simulink model "IEEE80211a"  (Simulink 10.0)
settings: Solver=VariableStepDiscrete  StartTime=0.0  StopTime=inf  RelTol=1e-3  EnableMultiTasking=on
PreLoadFcn:
  | load IEEE80211a_init;
undefined symbols (not defined in the file): hyst, j, magnitude, params, QAM, thres
libraries: simulink x27, IEEE80211a_lib x19, dspsigops x19, dspmtrx3 x19, dspsigattribs x15, dspmlti3 x10, dspstat3 x6, dspmathops x5, dspindex x3, dspsrcs4 x3, dspbuff3 x2, dspxfrm3 x2
(part 2 of 2)

== system IEEE80211a/Multipath channel/Multipath Rayleigh Fading Channel2 ==
  In : Inport
  Multipath Fading Channel : Subsystem  mask(Multipath Fading Channel){Fd=Fd, LOSFd=0, K=0, simTs=simTs, delayVec=delayVec, gainVecdB=gainVecdB, normGain=on, Seed=Seed}
      mask prompts: Fd "Doppler frequency (Hz):"; LOSFd "Line-of-sight Doppler frequency (Hz):"; K "K-factor:"; simTs "Sample time (sec):"; delayVec "Delay vector (sec):"; gainVecdB "Gain vector (dB):"; normGain "Normalize gain vector to 0 dB overall gain"; Seed "Initial seed:"
      mask help:
      | Multipath fading channel for complex baseband signals.
      |
      | Multiplies the input signal with samples of a complex random process. The spectrum of the random process is given by the Jakes PSD, where the Doppler frequency parameter determines the maximum Doppler frequency. The K-factor parameter specifies the linear ratio of power in the direct path to the diffuse power.
      |
      | The number of paths equals the length of either the 'Delay vector' or 'Gain vector' parameters.
      mask init:
      | [ecode,emsg,params] = commblkfadingchan2(gcb,Fd,LOSFd,K,simTs,delayVec,gainVecdB,normGain,Seed);
      | if(ecode==1)
      |     error(emsg);
      | elseif(ecode==2)
      |     warning(emsg);
      | end;
      mask Display:
      | plot(0,0,100,100,[05 15 10 10 05 10 18 14 13 7.5 13 41 44 47 50 53 57 59 100-[13 7.5 13 14 18 10 5 10 10 15 5]],[70 70 70 85 92 85 79 82 90 88.5 90 90 87 93 87 93 87 90 90 88.5 90 82 79 85 92 85 70 70 70]);
      | disp('Multipath\nFading')
  Out : Outport
  wires:
  Multipath Fading Channel/1(Out) -> Out/1
  In/1 -> Multipath Fading Channel/1(In)

== system IEEE80211a/Multipath channel/invdB1 ==
  gain : Inport
  Gain : Gain  Gain=-0.1  SaturateOnIntegerOverflow=on  OutDataTypeStr=Inherit: Same as input  ParamDataTypeStr=Inherit: Same as input
  Math Function : Math  Operator=10^u  SaturateOnIntegerOverflow=on
  dB : Outport
  wires:
  Math Function/1 -> dB/1
  gain/1 -> Gain/1
  Gain/1 -> Math Function/1

== system IEEE80211a/PER calculation/Bit indices ==
  mode : Inport
  delay : Inport  Port=2
  Constant : Constant  Value=(1:max(params.bitsPerBlock)).'  VectorParams1D=off
  Product : Product  Inputs=3  SaturateOnIntegerOverflow=on  OutDataTypeStr=Inherit: Same as first input
  Relational Operator1 : RelationalOperator  Operator=<=  OutDataTypeStr=float('double')  RndMeth=Nearest  InputSameDT=on
  Relational Operator2 : RelationalOperator  Operator=>  OutDataTypeStr=float('double')  RndMeth=Nearest  InputSameDT=on
  bits per block : IEEE80211a_lib/Select value  vector=params.bitsPerBlock.'
  sel : Outport
  wires:
  Relational Operator1/1 -> Product/2
  Relational Operator2/1 -> Product/3
  delay/1 -> Relational Operator2/2
  Product/1 -> sel/1
  bits per block/1 -> Relational Operator1/2
  Constant/1 -> Relational Operator1/1, Relational Operator2/1, Product/1
  mode/1 -> bits per block/1

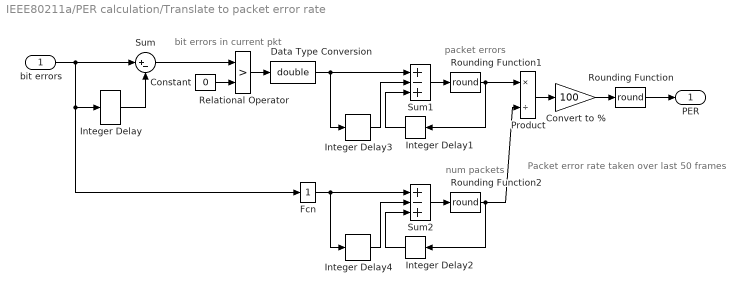
== system IEEE80211a/PER calculation/Translate to packet error rate ==
  note: Packet error rate taken over last 50 frames
  note: bit errors in
      | current pkt
  note: packet errors
  note: num packets
  bit errors : Inport
  Constant : Constant  Value=0
  Convert to % : Gain  Gain=100  SaturateOnIntegerOverflow=on  OutDataTypeStr=Inherit: Same as input  ParamDataTypeStr=Inherit: Same as input
  Data Type Conversion : DataTypeConversion  OutDataTypeStr=double  SaturateOnIntegerOverflow=on  RndMeth=Zero
  Fcn : Fcn  Expr=1
  Integer Delay : dspsigops/Integer Delay  delay=1  ic=0  reset_popup=None
      settings: SourceProductName=DSP System Toolbox  SourceProductBaseCode=DS
  Integer Delay1 : dspsigops/Integer Delay  delay=1  ic=0  reset_popup=None
      settings: SourceProductName=DSP System Toolbox  SourceProductBaseCode=DS
  Integer Delay2 : dspsigops/Integer Delay  delay=1  ic=0  reset_popup=None
      settings: SourceProductName=DSP System Toolbox  SourceProductBaseCode=DS
  Integer Delay3 : dspsigops/Integer Delay  delay=50  ic=0  reset_popup=None
      settings: SourceProductName=DSP System Toolbox  SourceProductBaseCode=DS
  Integer Delay4 : dspsigops/Integer Delay  delay=50  ic=0  reset_popup=None
      settings: SourceProductName=DSP System Toolbox  SourceProductBaseCode=DS
  Product : Product  Inputs=*/  SaturateOnIntegerOverflow=on  OutDataTypeStr=Inherit: Same as first input
  Relational Operator : RelationalOperator  Operator=>  RndMeth=Nearest
  Rounding Function : Rounding  Operator=round
  Rounding Function1 : Rounding  Operator=round
  Rounding Function2 : Rounding  Operator=round
  Sum : Sum  Inputs=|+-  SaturateOnIntegerOverflow=on
  Sum1 : Sum  Inputs=+-+  SaturateOnIntegerOverflow=on
  Sum2 : Sum  Inputs=+-+  SaturateOnIntegerOverflow=on
  PER : Outport
  wires:
  Rounding Function2/1 -> Integer Delay2/1, Product/2
  Rounding Function1/1 -> Integer Delay1/1, Product/1
  Rounding Function/1 -> PER/1
  Sum1/1 -> Rounding Function1/1
  Integer Delay1/1 -> Sum1/3
  Integer Delay3/1 -> Sum1/2
  Data Type Conversion/1 -> Sum1/1, Integer Delay3/1
  Integer Delay2/1 -> Sum2/3
  Integer Delay4/1 -> Sum2/2
  Sum2/1 -> Rounding Function2/1
  bit errors/1 -> Fcn/1, Integer Delay/1, Sum/1
  Convert to %/1 -> Rounding Function/1
  Product/1 -> Convert to %/1
  Fcn/1 -> Integer Delay4/1, Sum2/1
  Constant/1 -> Relational Operator/2
  Relational Operator/1 -> Data Type Conversion/1
  Sum/1 -> Relational Operator/1
  Integer Delay/1 -> Sum/2

== system IEEE80211a/Multipath channel/Multipath Rayleigh Fading Channel1/Multipath Fading Channel ==
  In : Inport
  Combine Paths : dspmtrx3/Matrix Sum  Dim=Rows
      settings: SourceProductName=DSP System Toolbox  SourceProductBaseCode=DS
  Fading Profile : Subsystem
      mask Display: disp('Fading\nProfile')
  Multiple Delayed Signals : Subsystem  mask(Multiple Delayed Signals){delayVector=params.sampleDelayVec, Ts=simTs}
      mask prompts: delayVector "Path delay vector:"; Ts "Sample time (sec):"
      mask init:
      | nPaths = length(delayVector);
      | maxDelay = ceil(max(delayVector))+1;
      mask Display: disp('Multiple\ndelayed signals');
  Multiply with  back propagation : Subsystem  mask(Multiply with back propagation){propTarget=Input 2, Ts=simTs, numChan=params.nPaths}
      mask prompts: propTarget "Propagation target:"; Ts "Sample time:"; numChan "Number of channels:"
      mask help:
      | Perform multiplication of the two input signals.
      |
      | The width and complexity of the output and the port not targeted for propagation must be identical. The width and complexity of the port targeted for propagation is set to that of the other input.
      |
      | The block sample time is the product of the number of samples per frame and the sample time parameter.
      mask TypeOptions propTarget: Input 1 | Input 2
      mask Display: disp('Multiply\nwith prop');
  Out : Outport
  wires:
  Combine Paths/1 -> Out/1
  Multiply with  back propagation/1(Out1) -> Combine Paths/1
  In/1 -> Multiple Delayed Signals/1(In)
  Fading Profile/1(Out) -> Multiply with  back propagation/2(In2)
  Multiple Delayed Signals/1(Out) -> Multiply with  back propagation/1(In1)

== system IEEE80211a/Multipath channel/Multipath Rayleigh Fading Channel2/Multipath Fading Channel ==
  In : Inport
  Combine Paths : dspmtrx3/Matrix Sum  Dim=Rows
      settings: SourceProductName=DSP System Toolbox  SourceProductBaseCode=DS
  Fading Profile : Subsystem
      mask Display: disp('Fading\nProfile')
  Multiple Delayed Signals : Subsystem  mask(Multiple Delayed Signals){delayVector=params.sampleDelayVec, Ts=simTs}
      mask prompts: delayVector "Path delay vector:"; Ts "Sample time (sec):"
      mask init:
      | nPaths = length(delayVector);
      | maxDelay = ceil(max(delayVector))+1;
      mask Display: disp('Multiple\ndelayed signals');
  Multiply with  back propagation : Subsystem  mask(Multiply with back propagation){propTarget=Input 2, Ts=simTs, numChan=params.nPaths}
      mask prompts: propTarget "Propagation target:"; Ts "Sample time:"; numChan "Number of channels:"
      mask help:
      | Perform multiplication of the two input signals.
      |
      | The width and complexity of the output and the port not targeted for propagation must be identical. The width and complexity of the port targeted for propagation is set to that of the other input.
      |
      | The block sample time is the product of the number of samples per frame and the sample time parameter.
      mask TypeOptions propTarget: Input 1 | Input 2
      mask Display: disp('Multiply\nwith prop');
  Out : Outport
  wires:
  Combine Paths/1 -> Out/1
  Multiply with  back propagation/1(Out1) -> Combine Paths/1
  In/1 -> Multiple Delayed Signals/1(In)
  Fading Profile/1(Out) -> Multiply with  back propagation/2(In2)
  Multiple Delayed Signals/1(Out) -> Multiply with  back propagation/1(In1)

== system IEEE80211a/Multipath channel/Multipath Rayleigh Fading Channel1/Multipath Fading Channel/Fading Profile ==
  Rebuffer with  Input Trigger : Subsystem  mask(Rebuffer with Input Trigger){startSample=params.startDelay, numChan=params.nPaths, inputWidthMode=Based on output width, inputWidth=params.intFactor, inputWidthMin=params.intFactor, inputWidthStep=params.intFactor}
      mask prompts: startSample "Start delay:"; numChan "Number of channels:"; inputWidthMode "Input width mode:"; inputWidth "Input width (per channel):"; inputWidthMin "Minimum input width (per channel):"; inputWidthStep "Input width step size (per channel):"
      mask help: This block inherits the input and output port widths and complexity and the output sample time. The input must be from a function call subsystem. The block generates a function call trigger on port 1 when ever data is required. and outputs the buffered input data on port 2.
      mask init:
      | s = commblktriggeredbuffer(gcb,'init',{});
      mask TypeOptions inputWidthMode: Inherit | Specify | Based on output width
      mask Callback inputWidthMode: commblktriggeredbuffer(gcb,'InputWidthMode');
      mask Display:
      | disp('Rebuffer\nwith trigger');
      | port_label('input',s.i1,s.i1s);
      | port_label('output',s.o1,s.o1s);
      | port_label('output',s.o2,s.o2s);
  Rician Channel  Effects : Subsystem  mask(Ricean Channel Effects){Doppler=params.LOSFd, K=params.K, opPower=params.gainVecLin, Ts=simTs, numChan=params.nPaths}
      mask prompts: Doppler "Line-of-sight Doppler frequency (Hz):"; K "K-factor"; opPower "Required output power (Watts):"; Ts "Sample time (s):"; numChan "Number of channels:"
      mask help: Add a complex phasor to the unity variance complex input to produce Rician channel effects. The Doppler frequency parameter determines frequency of the complex phasor.
      mask Display: disp('Rician\nChannel')
  Triggered Rayleigh Profile : Subsystem  TreatAsAtomicUnit=on
  Out : Outport
  wires:
  Rebuffer with  Input Trigger/2(Out2) -> Rician Channel  Effects/1(In)
  Rician Channel  Effects/1(Out) -> Out/1
  Rebuffer with  Input Trigger/1(Out1) -> Triggered Rayleigh Profile/Trigger
  Triggered Rayleigh Profile/1(Out) -> Rebuffer with  Input Trigger/1(In1)

== system IEEE80211a/Multipath channel/Multipath Rayleigh Fading Channel1/Multipath Fading Channel/Multiple Delayed Signals ==
  In : Inport
  Check Signal Attributes : dspsigattribs/Check Signal Attributes  SigAttribCheckMethod=Does not match attributes exactly  Complexity=Ignore  Frame=Ignore  DimsCheckMethod=Is...  Dimensions=Column vector (2-D) or scalar  DatatypeCheckMethod=Ignore  DatatypeGeneral=Boolean  DtypeFloatSpecific=Any floating-point  DtypeFixedSpecific=Any fixed-point  DtypeIntSpecific=Any integer  SampleMode=Ignore
      settings: SourceProductName=DSP System Toolbox  SourceProductBaseCode=DS
  Constant2 : Constant  Value=[delayVector(:)]'  VectorParams1D=off
  Constant3 : Constant  Value=ones(1,nPaths)  VectorParams1D=off
  Permute Matrix : dspmtrx3/Permute Matrix  mode=Columns  ZeroOneIdxMode=One-based  errmode=Clip Index  checkDims=off
      settings: SourceProductName=DSP System Toolbox  SourceProductBaseCode=DS
  Variable Fractional Delay : dspsigops/Variable Fractional Delay  mode=FIR Interpolation  dmax=maxDelay  L=6  R=10  alpha=1  ic=0
      settings: SourceProductName=DSP System Toolbox  SourceProductBaseCode=DS
  Out : Outport
  wires:
  In/1 -> Check Signal Attributes/1
  Constant2/1 -> Variable Fractional Delay/2
  Constant3/1 -> Permute Matrix/2
  Permute Matrix/1 -> Variable Fractional Delay/1
  Check Signal Attributes/1 -> Permute Matrix/1
  Variable Fractional Delay/1 -> Out/1

== system IEEE80211a/Multipath channel/Multipath Rayleigh Fading Channel1/Multipath Fading Channel/Multiply with  back propagation ==
  In1 : Inport
  In2 : Inport  Port=2
  S-Function : S-Function  FunctionName=scommultwithprop2  Parameters=propTarget, Ts, numChan  SFunctionDeploymentMode=off  EnableBusSupport=off
  Out1 : Outport
  wires:
  In2/1 -> S-Function/2
  In1/1 -> S-Function/1
  S-Function/1 -> Out1/1

== system IEEE80211a/Multipath channel/Multipath Rayleigh Fading Channel2/Multipath Fading Channel/Fading Profile ==
  Rebuffer with  Input Trigger : Subsystem  mask(Rebuffer with Input Trigger){startSample=params.startDelay, numChan=params.nPaths, inputWidthMode=Based on output width, inputWidth=params.intFactor, inputWidthMin=params.intFactor, inputWidthStep=params.intFactor}
      mask prompts: startSample "Start delay:"; numChan "Number of channels:"; inputWidthMode "Input width mode:"; inputWidth "Input width (per channel):"; inputWidthMin "Minimum input width (per channel):"; inputWidthStep "Input width step size (per channel):"
      mask help: This block inherits the input and output port widths and complexity and the output sample time. The input must be from a function call subsystem. The block generates a function call trigger on port 1 when ever data is required. and outputs the buffered input data on port 2.
      mask init:
      | s = commblktriggeredbuffer(gcb,'init',{});
      mask TypeOptions inputWidthMode: Inherit | Specify | Based on output width
      mask Callback inputWidthMode: commblktriggeredbuffer(gcb,'InputWidthMode');
      mask Display:
      | disp('Rebuffer\nwith trigger');
      | port_label('input',s.i1,s.i1s);
      | port_label('output',s.o1,s.o1s);
      | port_label('output',s.o2,s.o2s);
  Rician Channel  Effects : Subsystem  mask(Ricean Channel Effects){Doppler=params.LOSFd, K=params.K, opPower=params.gainVecLin, Ts=simTs, numChan=params.nPaths}
      mask prompts: Doppler "Line-of-sight Doppler frequency (Hz):"; K "K-factor"; opPower "Required output power (Watts):"; Ts "Sample time (s):"; numChan "Number of channels:"
      mask help: Add a complex phasor to the unity variance complex input to produce Rician channel effects. The Doppler frequency parameter determines frequency of the complex phasor.
      mask Display: disp('Rician\nChannel')
  Triggered Rayleigh Profile : Subsystem  TreatAsAtomicUnit=on
  Out : Outport
  wires:
  Rebuffer with  Input Trigger/2(Out2) -> Rician Channel  Effects/1(In)
  Rician Channel  Effects/1(Out) -> Out/1
  Rebuffer with  Input Trigger/1(Out1) -> Triggered Rayleigh Profile/Trigger
  Triggered Rayleigh Profile/1(Out) -> Rebuffer with  Input Trigger/1(In1)

== system IEEE80211a/Multipath channel/Multipath Rayleigh Fading Channel2/Multipath Fading Channel/Multiple Delayed Signals ==
  In : Inport
  Check Signal Attributes : dspsigattribs/Check Signal Attributes  SigAttribCheckMethod=Does not match attributes exactly  Complexity=Ignore  Frame=Ignore  DimsCheckMethod=Is...  Dimensions=Column vector (2-D) or scalar  DatatypeCheckMethod=Ignore  DatatypeGeneral=Boolean  DtypeFloatSpecific=Any floating-point  DtypeFixedSpecific=Any fixed-point  DtypeIntSpecific=Any integer  SampleMode=Ignore
      settings: SourceProductName=DSP System Toolbox  SourceProductBaseCode=DS
  Constant2 : Constant  Value=[delayVector(:)]'  VectorParams1D=off
  Constant3 : Constant  Value=ones(1,nPaths)  VectorParams1D=off
  Permute Matrix : dspmtrx3/Permute Matrix  mode=Columns  ZeroOneIdxMode=One-based  errmode=Clip Index  checkDims=off
      settings: SourceProductName=DSP System Toolbox  SourceProductBaseCode=DS
  Variable Fractional Delay : dspsigops/Variable Fractional Delay  mode=FIR Interpolation  dmax=maxDelay  L=6  R=10  alpha=1  ic=0
      settings: SourceProductName=DSP System Toolbox  SourceProductBaseCode=DS
  Out : Outport
  wires:
  In/1 -> Check Signal Attributes/1
  Constant2/1 -> Variable Fractional Delay/2
  Constant3/1 -> Permute Matrix/2
  Permute Matrix/1 -> Variable Fractional Delay/1
  Check Signal Attributes/1 -> Permute Matrix/1
  Variable Fractional Delay/1 -> Out/1

== system IEEE80211a/Multipath channel/Multipath Rayleigh Fading Channel2/Multipath Fading Channel/Multiply with  back propagation ==
  In1 : Inport
  In2 : Inport  Port=2
  S-Function : S-Function  FunctionName=scommultwithprop2  Parameters=propTarget, Ts, numChan  SFunctionDeploymentMode=off  EnableBusSupport=off
  Out1 : Outport
  wires:
  In2/1 -> S-Function/2
  In1/1 -> S-Function/1
  S-Function/1 -> Out1/1

== system IEEE80211a/Multipath channel/Multipath Rayleigh Fading Channel1/Multipath Fading Channel/Fading Profile/Rebuffer with  Input Trigger ==
  In1 : Inport
  S-Function : S-Function  FunctionName=scomtrigbuff2  Parameters=startSample, numChan, inputWidthMode, inputWidth, inputWidthMin, inputWidthStep  SFunctionDeploymentMode=off  EnableBusSupport=off
  Out1 : Outport
  Out2 : Outport  Port=2
  wires:
  S-Function/1 -> Out1/1
  S-Function/2 -> Out2/1
  In1/1 -> S-Function/1

== system IEEE80211a/Multipath channel/Multipath Rayleigh Fading Channel1/Multipath Fading Channel/Fading Profile/Rician Channel  Effects ==
  In : Inport
  S-Function : S-Function  FunctionName=scomricianlos2  Parameters=Doppler,K,opPower,Ts,numChan  SFunctionDeploymentMode=off  EnableBusSupport=off
  Out : Outport
  wires:
  In/1 -> S-Function/1
  S-Function/1 -> Out/1

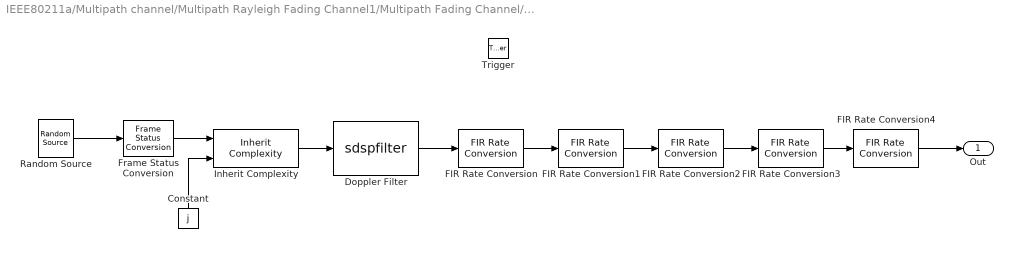
== system IEEE80211a/Multipath channel/Multipath Rayleigh Fading Channel1/Multipath Fading Channel/Fading Profile/Triggered Rayleigh Profile ==
  Trigger : TriggerPort  TriggerType=function-call  VariantControl=(inherit)
  Constant : Constant  Value=j
  Doppler Filter : S-Function  AncestorBlock=dsparch4/Digital Filter  FunctionName=sdspfilter  Parameters=a.CoeffsFromMask, a.FilterType, a.FilterStruct, a.FilterPerSample, a.CoeffsNormalized, a.Coeff1, a.Coeff2, a.IC,1  SFunctionDeploymentMode=off  EnableBusSupport=off  mask(Digital Filter){TypePopup=IIR (poles & zeros), IIRFiltStruct=Biquad direct form II transposed (SOS), AllPoleFiltStruct=Direct form, FIRFiltStruct=Direct form, CoeffSource=Specify via dialog, NumCoeffs=[1 2], DenCoeffs=[1 0.1], BiQuadCoeffs=params.dopplerSos, LatticeCoeffs=[0.2 0.4], denIgnore=on, FiltPerSampPopup=One filter per frame, IC=0, ICnum=0, ICden=0}
      mask prompts: TypePopup "Transfer function type:"; IIRFiltStruct "Filter structure:"; AllPoleFiltStruct "Filter structure:"; FIRFiltStruct "Filter structure:"; CoeffSource "Coefficient source:"; NumCoeffs "Numerator coefficients:"; DenCoeffs "Denominator coefficients:"; BiQuadCoeffs "SOS matrix (Mx6):"; LatticeCoeffs "Reflection coefficients:"; denIgnore "First denominator coefficient = 1, remove 1/a0 term in the structure"; FiltPerSampPopup "Coefficient update rate:"; IC "Initial conditions:"; ICnum "Initial conditions on zeros side:"; ICden "Initial conditions on poles side:"
      mask help:
      | Independently filter each channel of the input over time using a specified digital filter implementation.  Filter coefficients can be specified using either tunable mask dialog parameters or separate input ports (useful for time-varying coefficients).
      |
      | Time-varying coefficients are supported at one of two possible rates of coefficient update in frame-based processing.  The coefficients can update at a rate of one filter per frame (i.e. they stay constant for the duration of an input frame and change for the next frame).  Or, the coefficients can update at a rate of one filter per sample (i.e. they change with every sample in the input frame).
      mask init:
      | s = dspblkfilter('icon');
      | a = dspblkfilter('init');
      mask Help: web(dspbhelp);
      mask TypeOptions TypePopup: IIR (poles & zeros) | IIR (all poles) | FIR (all zeros)
      mask Callback TypePopup: dspblkfilter('dynamic');
      mask TypeOptions IIRFiltStruct: Direct form I | Direct form I transposed | Direct form II | Direct form II transposed | Biquad direct form II transposed (SOS)
      mask Callback IIRFiltStruct: dspblkfilter('dynamic');
      mask TypeOptions AllPoleFiltStruct: Direct form | Direct form transposed | Lattice AR
      mask Callback AllPoleFiltStruct: dspblkfilter('dynamic');
      mask TypeOptions FIRFiltStruct: Direct form | Direct form transposed | Lattice MA
      mask Callback FIRFiltStruct: dspblkfilter('dynamic');
      mask TypeOptions CoeffSource: Specify via dialog | Input port(s)
      mask Callback CoeffSource: dspblkfilter('dynamic');
      mask TypeOptions FiltPerSampPopup: One filter per frame | One filter per sample
      mask Display:
      | text(0.5,0.85,s.icon,'horiz','center');
      | plot(s.x, s.y);
      | port_label('input',s.i1,s.s1);
      | port_label('input',s.i2,s.s2);
      | port_label('input',1,s.in);
      | port_label('output',1,s.out);
  FIR Rate Conversion : dspmlti3/FIR Rate Conversion  L=params.interp1  h=params.rc1Num  M=params.decim1
      settings: SourceProductName=DSP System Toolbox  SourceProductBaseCode=DS
  FIR Rate Conversion1 : dspmlti3/FIR Rate Conversion  L=params.interp2  h=params.rc2Num  M=params.decim2
      settings: SourceProductName=DSP System Toolbox  SourceProductBaseCode=DS
  FIR Rate Conversion2 : dspmlti3/FIR Rate Conversion  L=params.interp3  h=params.rc3Num  M=params.decim3
      settings: SourceProductName=DSP System Toolbox  SourceProductBaseCode=DS
  FIR Rate Conversion3 : dspmlti3/FIR Rate Conversion  L=params.interp4  h=params.rc4Num  M=params.decim4
      settings: SourceProductName=DSP System Toolbox  SourceProductBaseCode=DS
  FIR Rate Conversion4 : dspmlti3/FIR Rate Conversion  L=params.interp5  h=params.rc5Num  M=params.decim5
      settings: SourceProductName=DSP System Toolbox  SourceProductBaseCode=DS
  Frame Status Conversion : dspsigattribs/Frame Status Conversion  growRefPort=off  outframe=Frame-based
      settings: SourceProductName=DSP System Toolbox  SourceProductBaseCode=DS
  Inherit Complexity : dspsigattribs/Inherit Complexity
      settings: SourceProductName=DSP System Toolbox  SourceProductBaseCode=DS
  Random Source : dspsrcs4/Random Source  SrcType=Gaussian  NormMethod=Ziggurat  CltLength=12  Min=0  Max=1  Mean=0  Var=1  RepMode=Specify seed  Seed=params.Seed  Inherit=on  SampMode=Discrete  SampTime=1  SampFrame=1  DataType=Double  OutComplex=Real
  Out : Outport
  wires:
  FIR Rate Conversion4/1 -> Out/1
  FIR Rate Conversion1/1 -> FIR Rate Conversion2/1
  Doppler Filter/1 -> FIR Rate Conversion/1
  FIR Rate Conversion/1 -> FIR Rate Conversion1/1
  Inherit Complexity/1 -> Doppler Filter/1
  Constant/1 -> Inherit Complexity/2
  Random Source/1 -> Frame Status Conversion/1
  Frame Status Conversion/1 -> Inherit Complexity/1
  FIR Rate Conversion2/1 -> FIR Rate Conversion3/1
  FIR Rate Conversion3/1 -> FIR Rate Conversion4/1

== system IEEE80211a/Multipath channel/Multipath Rayleigh Fading Channel2/Multipath Fading Channel/Fading Profile/Rebuffer with  Input Trigger ==
  In1 : Inport
  S-Function : S-Function  FunctionName=scomtrigbuff2  Parameters=startSample, numChan, inputWidthMode, inputWidth, inputWidthMin, inputWidthStep  SFunctionDeploymentMode=off  EnableBusSupport=off
  Out1 : Outport
  Out2 : Outport  Port=2
  wires:
  S-Function/1 -> Out1/1
  S-Function/2 -> Out2/1
  In1/1 -> S-Function/1

== system IEEE80211a/Multipath channel/Multipath Rayleigh Fading Channel2/Multipath Fading Channel/Fading Profile/Rician Channel  Effects ==
  In : Inport
  S-Function : S-Function  FunctionName=scomricianlos2  Parameters=Doppler,K,opPower,Ts,numChan  SFunctionDeploymentMode=off  EnableBusSupport=off
  Out : Outport
  wires:
  In/1 -> S-Function/1
  S-Function/1 -> Out/1

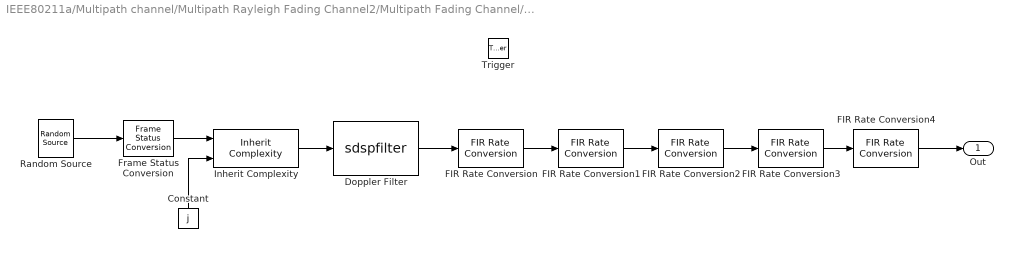
== system IEEE80211a/Multipath channel/Multipath Rayleigh Fading Channel2/Multipath Fading Channel/Fading Profile/Triggered Rayleigh Profile ==
  Trigger : TriggerPort  TriggerType=function-call  VariantControl=(inherit)
  Constant : Constant  Value=j
  Doppler Filter : S-Function  AncestorBlock=dsparch4/Digital Filter  FunctionName=sdspfilter  Parameters=a.CoeffsFromMask, a.FilterType, a.FilterStruct, a.FilterPerSample, a.CoeffsNormalized, a.Coeff1, a.Coeff2, a.IC,1  SFunctionDeploymentMode=off  EnableBusSupport=off  mask(Digital Filter){TypePopup=IIR (poles & zeros), IIRFiltStruct=Biquad direct form II transposed (SOS), AllPoleFiltStruct=Direct form, FIRFiltStruct=Direct form, CoeffSource=Specify via dialog, NumCoeffs=[1 2], DenCoeffs=[1 0.1], BiQuadCoeffs=params.dopplerSos, LatticeCoeffs=[0.2 0.4], denIgnore=on, FiltPerSampPopup=One filter per frame, IC=0, ICnum=0, ICden=0}
      mask prompts: TypePopup "Transfer function type:"; IIRFiltStruct "Filter structure:"; AllPoleFiltStruct "Filter structure:"; FIRFiltStruct "Filter structure:"; CoeffSource "Coefficient source:"; NumCoeffs "Numerator coefficients:"; DenCoeffs "Denominator coefficients:"; BiQuadCoeffs "SOS matrix (Mx6):"; LatticeCoeffs "Reflection coefficients:"; denIgnore "First denominator coefficient = 1, remove 1/a0 term in the structure"; FiltPerSampPopup "Coefficient update rate:"; IC "Initial conditions:"; ICnum "Initial conditions on zeros side:"; ICden "Initial conditions on poles side:"
      mask help:
      | Independently filter each channel of the input over time using a specified digital filter implementation.  Filter coefficients can be specified using either tunable mask dialog parameters or separate input ports (useful for time-varying coefficients).
      |
      | Time-varying coefficients are supported at one of two possible rates of coefficient update in frame-based processing.  The coefficients can update at a rate of one filter per frame (i.e. they stay constant for the duration of an input frame and change for the next frame).  Or, the coefficients can update at a rate of one filter per sample (i.e. they change with every sample in the input frame).
      mask init:
      | s = dspblkfilter('icon');
      | a = dspblkfilter('init');
      mask Help: web(dspbhelp);
      mask TypeOptions TypePopup: IIR (poles & zeros) | IIR (all poles) | FIR (all zeros)
      mask Callback TypePopup: dspblkfilter('dynamic');
      mask TypeOptions IIRFiltStruct: Direct form I | Direct form I transposed | Direct form II | Direct form II transposed | Biquad direct form II transposed (SOS)
      mask Callback IIRFiltStruct: dspblkfilter('dynamic');
      mask TypeOptions AllPoleFiltStruct: Direct form | Direct form transposed | Lattice AR
      mask Callback AllPoleFiltStruct: dspblkfilter('dynamic');
      mask TypeOptions FIRFiltStruct: Direct form | Direct form transposed | Lattice MA
      mask Callback FIRFiltStruct: dspblkfilter('dynamic');
      mask TypeOptions CoeffSource: Specify via dialog | Input port(s)
      mask Callback CoeffSource: dspblkfilter('dynamic');
      mask TypeOptions FiltPerSampPopup: One filter per frame | One filter per sample
      mask Display:
      | text(0.5,0.85,s.icon,'horiz','center');
      | plot(s.x, s.y);
      | port_label('input',s.i1,s.s1);
      | port_label('input',s.i2,s.s2);
      | port_label('input',1,s.in);
      | port_label('output',1,s.out);
  FIR Rate Conversion : dspmlti3/FIR Rate Conversion  L=params.interp1  h=params.rc1Num  M=params.decim1
      settings: SourceProductName=DSP System Toolbox  SourceProductBaseCode=DS
  FIR Rate Conversion1 : dspmlti3/FIR Rate Conversion  L=params.interp2  h=params.rc2Num  M=params.decim2
      settings: SourceProductName=DSP System Toolbox  SourceProductBaseCode=DS
  FIR Rate Conversion2 : dspmlti3/FIR Rate Conversion  L=params.interp3  h=params.rc3Num  M=params.decim3
      settings: SourceProductName=DSP System Toolbox  SourceProductBaseCode=DS
  FIR Rate Conversion3 : dspmlti3/FIR Rate Conversion  L=params.interp4  h=params.rc4Num  M=params.decim4
      settings: SourceProductName=DSP System Toolbox  SourceProductBaseCode=DS
  FIR Rate Conversion4 : dspmlti3/FIR Rate Conversion  L=params.interp5  h=params.rc5Num  M=params.decim5
      settings: SourceProductName=DSP System Toolbox  SourceProductBaseCode=DS
  Frame Status Conversion : dspsigattribs/Frame Status Conversion  growRefPort=off  outframe=Frame-based
      settings: SourceProductName=DSP System Toolbox  SourceProductBaseCode=DS
  Inherit Complexity : dspsigattribs/Inherit Complexity
      settings: SourceProductName=DSP System Toolbox  SourceProductBaseCode=DS
  Random Source : dspsrcs4/Random Source  SrcType=Gaussian  NormMethod=Ziggurat  CltLength=12  Min=0  Max=1  Mean=0  Var=1  RepMode=Specify seed  Seed=params.Seed  Inherit=on  SampMode=Discrete  SampTime=1  SampFrame=1  DataType=Double  OutComplex=Real
  Out : Outport
  wires:
  FIR Rate Conversion4/1 -> Out/1
  FIR Rate Conversion1/1 -> FIR Rate Conversion2/1
  Doppler Filter/1 -> FIR Rate Conversion/1
  FIR Rate Conversion/1 -> FIR Rate Conversion1/1
  Inherit Complexity/1 -> Doppler Filter/1
  Constant/1 -> Inherit Complexity/2
  Random Source/1 -> Frame Status Conversion/1
  Frame Status Conversion/1 -> Inherit Complexity/1
  FIR Rate Conversion2/1 -> FIR Rate Conversion3/1
  FIR Rate Conversion3/1 -> FIR Rate Conversion4/1

== stateflow chart Adaptive Modulation Control ==
  state Mod_BPSK_6Mbps
    entry: modIdx = 1;
    bitRate = 6;
  state Mod_BPSK2_9Mbps
    entry: modIdx = 2;
    bitRate = 9;
  state Mod_QPSK2_18Mbps
    entry: modIdx = 4;
    bitRate = 18;
  state Mod_QPSK_12Mbps
    entry: modIdx = 3;
    bitRate = 12;
  state Mod_64QAM2_54Mbps
    entry: modIdx = 8;
    bitRate = 54;
  state Mod_64QAM_48Mbps
    entry: modIdx = 7;
    bitRate = 48;
  note: The power of the Rx signal is compared against an array
      | of power thresholds in order to determine the corresponding
      | modulation as defined by the IEEE 802.11a specifications
  state Mod_16QAM_24Mbps
    entry: modIdx = 5;
    bitRate = 24;
  note: Finite State Machine that controls
      | the adaptive modulation scheme.
  state Mod_16QAM_36Mbps
    entry: modIdx = 6;
    bitRate = 36;
  Mod_BPSK2_9Mbps -> Mod_BPSK_6Mbps [order 2] : [snrEst<=thres[1]-hyst]
  Mod_BPSK_6Mbps -> Mod_BPSK2_9Mbps : [snrEst>thres[1]+hyst]
  Mod_QPSK_12Mbps -> Mod_BPSK2_9Mbps [order 2] : [snrEst<=thres[2]-hyst]
  Mod_BPSK2_9Mbps -> Mod_QPSK_12Mbps [order 1] : [snrEst>thres[2]+hyst]
  Mod_QPSK2_18Mbps -> Mod_QPSK_12Mbps [order 2] : [snrEst<=thres[3]-hyst]
  Mod_QPSK_12Mbps -> Mod_QPSK2_18Mbps [order 1] : [snrEst>thres[3]+hyst]
  (default) -> Mod_QPSK2_18Mbps
  Mod_16QAM_24Mbps -> Mod_QPSK2_18Mbps [order 2] : [snrEst<=thres[4]-hyst]
  Mod_QPSK2_18Mbps -> Mod_16QAM_24Mbps [order 1] : [snrEst>thres[4]+hyst]
  Mod_16QAM_36Mbps -> Mod_16QAM_24Mbps [order 2] : [snrEst<=thres[5]-hyst]
  Mod_16QAM_24Mbps -> Mod_16QAM_36Mbps [order 1] : [snrEst>thres[5]+hyst]
  Mod_64QAM_48Mbps -> Mod_16QAM_36Mbps [order 2] : [snrEst<=thres[6]-hyst]
  Mod_16QAM_36Mbps -> Mod_64QAM_48Mbps [order 1] : [snrEst>thres[6]+hyst]
  Mod_64QAM2_54Mbps -> Mod_64QAM_48Mbps : [snrEst<=thres[7]-hyst]
  Mod_64QAM_48Mbps -> Mod_64QAM2_54Mbps [order 1] : [snrEst>thres[7]+hyst]
  data: snrEst input double; modIdx output double; thres local double size=[1 7] =thres; hyst local double =hyst; bitRate output double
